simulink model "HIL"  (R2025b)
settings: Solver=FixedStepAuto  StartTime=0.0  StopTime=10.0  FixedStep=0.01  RelTol=1e-3
settings Model: Creator=Adham  LastModifiedBy=Adham
settings RTWCC: CustomInclude=|
  | C:\ProgramData\MATLAB\SupportPackages\R2025b\aCLI\data\packages\esp32\hardware\esp32\2.0.11\libraries\Wire\src
  | core\inc
  | platform\inc
settings RTWCC: CustomSource=|
  | C:\ProgramData\MATLAB\SupportPackages\R2025b\aCLI\data\packages\esp32\hardware\esp32\2.0.11\libraries\Wire\src\Wire.cpp
  | core\src\vl53l0x_api.cpp
  | core\src\vl53l0x_api_calibration.cpp
  | core\src\vl53l0x_api_core.cpp
  | core\src\vl53l0x_api_ranging.cpp
  | core\src\vl53l0x_api_strings.cpp
  | platform\src\vl53l0x_platform.cpp
  | Adafruit_VL53L0X.cpp

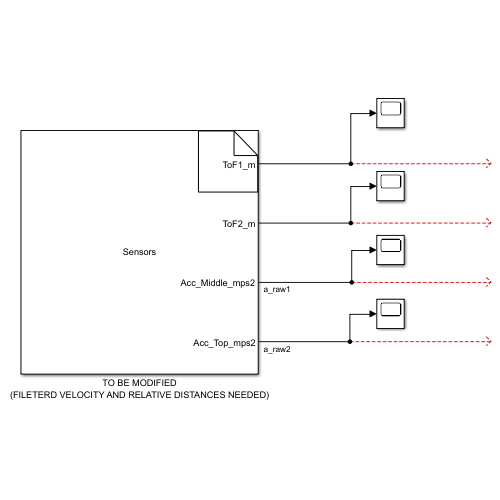
[thumbnail: Simulink's stored preview of the top-level diagram]
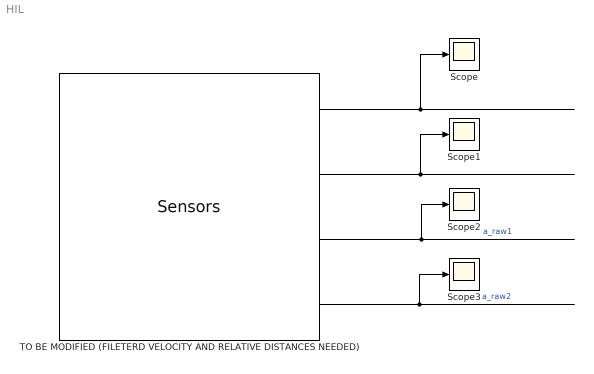
== system HIL ==
  Scope{,1..3} (4 alike) : Scope
      Scope2 settings: DataLoggingVariableName=ScopeData2
      Scope3 settings: DataLoggingVariableName=ScopeData3
  TO BE MODIFIED (FILETERD VELOCITY AND RELATIVE DISTANCES NEEDED) : S-Function  FunctionName=Sensors  SFunctionModules=Sensors_wrapper.cpp  SFunctionDeploymentMode=off  EnableBusSupport=off  mask(S-Function Builder){}
      mask help: Simulink:masks:SFunctionBuilder_MD
      mask init:
      | val = [[.9  0.75 0.75 1 1 .9 .9 1]',[1 1 0.75 0.75 .9 .9 1 .9]'];try , sys = get_param(gcb,'SfunBuilderFcnName');if isempty(sys), sys = get_param(gcb,'FunctionName'); end,catch, sys = get_param(gcb,'FunctionName'); end
      settings: CopyFcn=set_param(gcbh,'LinkStatus','none')  OpenFcn=sfunctionwizard(gcbh)
      mask Display:
      | plot(val(:,1),val(:,2))
      | disp(sys)
      | port_label('output',1,sprintf('%s', 'ToF1\_m'),'interpreter','tex')
      | port_label('output',2,sprintf('%s', 'ToF2\_m'),'interpreter','tex')
      | port_label('output',3,sprintf('%s', 'Acc\_Middle\_mps2'),'interpreter','tex')
      | port_label('output',4,sprintf('%s', 'Acc\_Top\_mps2'),'interpreter','tex')
  wires:
  TO BE MODIFIED (FILETERD VELOCITY AND RELATIVE DISTANCES NEEDED)/1 -> Scope/1
  TO BE MODIFIED (FILETERD VELOCITY AND RELATIVE DISTANCES NEEDED)/2 -> Scope1/1
  TO BE MODIFIED (FILETERD VELOCITY AND RELATIVE DISTANCES NEEDED)/3 -> Scope2/1  "a_raw1"
  TO BE MODIFIED (FILETERD VELOCITY AND RELATIVE DISTANCES NEEDED)/4 -> Scope3/1  "a_raw2"
